simulink model "PID_Dual_Robot_DC_model_no_vision_controller"  (R2015b)
settings: Solver=ode4  StartTime=0.0  StopTime=28  FixedStep=0.01  RelTol=1e-3
InitFcn:
  | Set_Parameter_sewing_DC_model_no_vision_controller
StopFcn:
  | DrawResult_Dual
values from neighbouring files (symbols this model uses):
  b = 0.1    [Set_Parameter.m]    (also in Set_Parameter_Single.m; Set_Parameter_line_circle.m; Set_Parameter_line_circle_DC_model_no_vision_controller.m; Set_Parameter_sewing_DC_model_no_vision_controller.m)
  D = [30,30,20,20,20,20,20,20]    [Set_Parameter.m]    (also in Set_Parameter_Single.m; Set_Parameter_line_circle.m; Set_Parameter_line_circle_DC_model_no_vision_controller.m; Set_Parameter_line_circle_no_vision_controller.m = [40,40,40,30,20,30,20,20])
  I = [10,10,5,5,5,2,2,2]    [Set_Parameter.m]    (also in Set_Parameter_Single.m; Set_Parameter_line_circle.m; Set_Parameter_line_circle_DC_model_no_vision_controller.m; Set_Parameter_line_circle_no_vision_controller.m = [5,5,5,2,2,2,1,1])
  IniJointAngle_L = theta_L    [Set_Parameter.m]    (also in Set_Parameter_Single.m; Set_Parameter_line_circle.m; Set_Parameter_line_circle_DC_model_no_vision_controller.m; Set_Parameter_line_circle_no_vision_controller.m)
  IniJointAngle_R = theta_R    [Set_Parameter.m]    (also in Set_Parameter_Single.m; Set_Parameter_line_circle.m; Set_Parameter_line_circle_DC_model_no_vision_controller.m; Set_Parameter_line_circle_no_vision_controller.m)
  J = [0.016,0.016,0.012,0.012,0.01,0.01,0.01]    [Set_Parameter.m]    (also in Set_Parameter_Single.m; Set_Parameter_line_circle.m; Set_Parameter_line_circle_DC_model_no_vision_controller.m; Set_Parameter_line_circle_no_vision_controller.m = [10,10,8,8,4,4,4])
  K = 0.01    [Set_Parameter.m]    (also in Set_Parameter_Single.m; Set_Parameter_line_circle.m; Set_Parameter_line_circle_DC_model_no_vision_controller.m; Set_Parameter_sewing_DC_model_no_vision_controller.m)
  L = 0.5    [Set_Parameter.m]    (also in Set_Parameter_Single.m; Set_Parameter_line_circle.m; Set_Parameter_line_circle_DC_model_no_vision_controller.m; Set_Parameter_sewing_DC_model_no_vision_controller.m)
  P = [60,60,50,50,30,30,20,20]    [Set_Parameter.m]    (also in Set_Parameter_Single.m; Set_Parameter_line_circle.m; Set_Parameter_line_circle_DC_model_no_vision_controller.m = [120,120,100,100,60,60,40,40]; Set_Parameter_line_circle_no_vision_controller.m = [350,100,300,150,50,100,20,20])
  R = R_z1x2y3(PoseAngle(1),PoseAngle(2),PoseAngle(3))    [IK_7DOF_FB7roll.m]    (also in Set_Parameter.m = 1; Set_Parameter_Single.m = 1; Set_Parameter_line_circle.m = 1; Set_Parameter_line_circle_DC_model_no_vision_controller.m = 1)
settings Model: Creator=User  LastModifiedBy=User

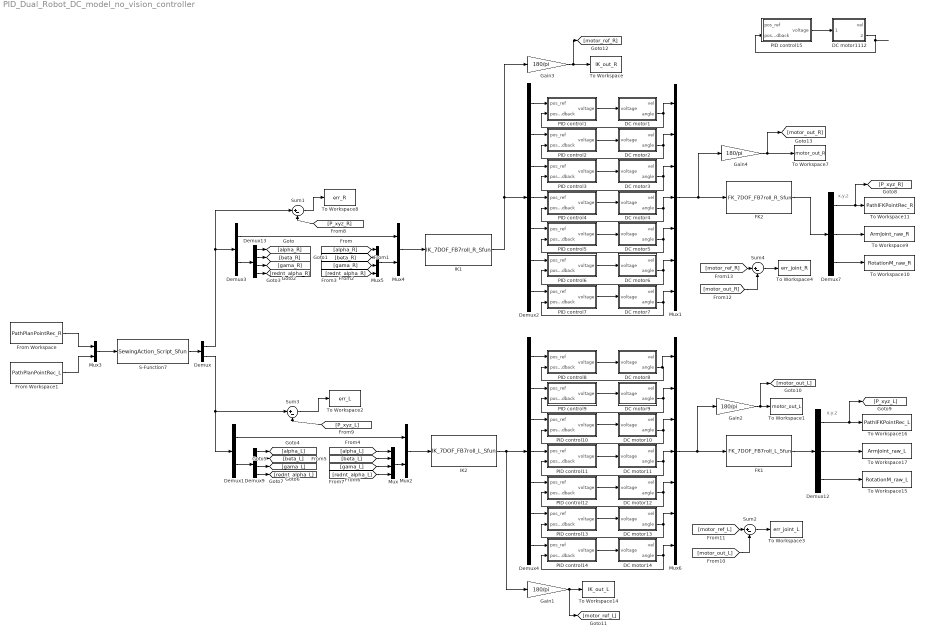
== system PID_Dual_Robot_DC_model_no_vision_controller ==
  note: x,y,z
  note: x,y,z
  DC motor1 : Subsystem
  DC motor10 : Subsystem
  DC motor11 : Subsystem
  DC motor1112 : Subsystem
  DC motor12 : Subsystem
  DC motor13 : Subsystem
  DC motor14 : Subsystem
  DC motor2 : Subsystem
  DC motor3 : Subsystem
  DC motor4 : Subsystem
  DC motor5 : Subsystem
  DC motor6 : Subsystem
  DC motor7 : Subsystem
  DC motor8 : Subsystem
  DC motor9 : Subsystem
  Demux : Demux  Outputs=[7,7]
  Demux1 : Demux  Outputs=[3,4]
  Demux12 : Demux  Outputs=[7,30,9]
  Demux13 : Demux
  Demux2 : Demux  Outputs=7
  Demux3 : Demux  Outputs=[3,4]
  Demux4 : Demux  Outputs=7
  Demux7 : Demux  Outputs=[7,30,9]
  Demux9 : Demux
  FK1 : S-Function  FunctionName=FK_7DOF_FB7roll_L_Sfun  SFunctionDeploymentMode=off  EnableBusSupport=off
  FK2 : S-Function  FunctionName=FK_7DOF_FB7roll_R_Sfun  SFunctionDeploymentMode=off  EnableBusSupport=off
  From Workspace : FromWorkspace  VariableName=PathPlanPointRec_R  SampleTime=0
  From Workspace1 : FromWorkspace  VariableName=PathPlanPointRec_L  SampleTime=0
  Gain{1..4} (4 alike) : Gain  Gain=180/pi
  IK1 : S-Function  FunctionName=IK_7DOF_FB7roll_R_Sfun  SFunctionDeploymentMode=off  EnableBusSupport=off
  IK2 : S-Function  FunctionName=IK_7DOF_FB7roll_L_Sfun  SFunctionDeploymentMode=off  EnableBusSupport=off
  Mux : Mux
  Mux1 : Mux  Inputs=7
  Mux2 : Mux  Inputs=[3,4]
  Mux3 : Mux  Inputs=[7,7]
  Mux4 : Mux  Inputs=[3,4]
  Mux5 : Mux
  Mux6 : Mux  Inputs=7
  PID control1 : Subsystem
  PID control10 : Subsystem
  PID control11 : Subsystem
  PID control12 : Subsystem
  PID control13 : Subsystem
  PID control14 : Subsystem
  PID control15 : Subsystem
  PID control2 : Subsystem
  PID control3 : Subsystem
  PID control4 : Subsystem
  PID control5 : Subsystem
  PID control6 : Subsystem
  PID control7 : Subsystem
  PID control8 : Subsystem
  PID control9 : Subsystem
  S-Function7 : S-Function  FunctionName=SewingAction_Script_Sfun  SFunctionDeploymentMode=off  EnableBusSupport=off
  Sum{1..4} (4 alike) : Sum  Inputs=|+-
  To Workspace : ToWorkspace  VariableName=IK_out_R  SaveFormat=Timeseries  SampleTime=-1
  To Workspace1 : ToWorkspace  VariableName=motor_out_L  SaveFormat=Timeseries  SampleTime=-1
  To Workspace10 : ToWorkspace  VariableName=RotationM_raw_R  SaveFormat=Timeseries  SampleTime=-1
  To Workspace11 : ToWorkspace  VariableName=PathIFKPointRec_R  SaveFormat=Timeseries  SampleTime=-1
  To Workspace14 : ToWorkspace  VariableName=IK_out_L  SaveFormat=Timeseries  SampleTime=-1
  To Workspace15 : ToWorkspace  VariableName=RotationM_raw_L  SaveFormat=Timeseries  SampleTime=-1
  To Workspace16 : ToWorkspace  VariableName=PathIFKPointRec_L  SaveFormat=Timeseries  SampleTime=-1
  To Workspace17 : ToWorkspace  VariableName=ArmJoint_raw_L  SaveFormat=Timeseries  SampleTime=-1
  To Workspace2 : ToWorkspace  VariableName=err_L  SaveFormat=Timeseries  SampleTime=-1
  To Workspace3 : ToWorkspace  VariableName=err_joint_L  SaveFormat=Timeseries  SampleTime=-1
  To Workspace4 : ToWorkspace  VariableName=err_joint_R  SaveFormat=Timeseries  SampleTime=-1
  To Workspace7 : ToWorkspace  VariableName=motor_out_R  SaveFormat=Timeseries  SampleTime=-1
  To Workspace8 : ToWorkspace  VariableName=err_R  SaveFormat=Timeseries  SampleTime=-1
  To Workspace9 : ToWorkspace  VariableName=ArmJoint_raw_R  SaveFormat=Timeseries  SampleTime=-1
  wires:
  Gain3/1 -> [motor_ref_R], To Workspace/1
  Gain4/1 -> [motor_out_R], To Workspace7/1
  Demux2/1 -> PID control1/1("pos_ref ")
  IK1/1 -> Demux2/1, Gain3/1
  Mux1/1 -> Gain4/1, FK2/1
  Mux4/1 -> IK1/1
  FK2/1 -> Demux7/1
  Demux7/1 -> To Workspace11/1, [P_xyz_R]
  Demux7/2 -> To Workspace9/1
  Demux7/3 -> To Workspace10/1
  S-Function7/1 -> Demux/1
  Demux/1 -> Sum1/1, Demux3/1
  Demux/2 -> Sum3/1, Demux1/1
  Demux9/1 -> [alpha_L]
  Demux9/2 -> [beta_L]
  Demux9/3 -> [gama_L]
  Demux9/4 -> [rednt_alpha_L]
  Demux1/2 -> Demux9/1
  [alpha_L] -> Mux/1
  [beta_L] -> Mux/2
  [gama_L] -> Mux/3
  [rednt_alpha_L] -> Mux/4
  Mux/1 -> Mux2/2
  Gain1/1 -> [motor_ref_L], To Workspace14/1
  IK2/1 -> Gain1/1, Demux4/1
  FK1/1 -> Demux12/1
  Demux12/2 -> To Workspace17/1
  Demux12/1 -> To Workspace16/1, [P_xyz_L]
  Demux12/3 -> To Workspace15/1
  Demux3/2 -> Demux13/1
  Demux13/2 -> [beta_R]
  Demux13/3 -> [gama_R]
  Demux13/4 -> [rednt_alpha_R]
  Gain2/1 -> [motor_out_L], To Workspace1/1
  Mux3/1 -> S-Function7/1
  From Workspace/1 -> Mux3/1
  From Workspace1/1 -> Mux3/2
  Mux2/1 -> IK2/1
  Mux5/1 -> Mux4/2
  [alpha_R] -> Mux5/1
  [beta_R] -> Mux5/2
  [gama_R] -> Mux5/3
  [rednt_alpha_R] -> Mux5/4
  Demux13/1 -> [alpha_R]
  PID control1/1(voltage) -> DC motor1/1(voltage)
  DC motor1/2(angle) -> Mux1/1, PID control1/2(pos_feedback)
  PID control2/1(voltage) -> DC motor2/1(voltage)
  DC motor2/2(angle) -> Mux1/2, PID control2/2(pos_feedback)
  Demux2/2 -> PID control2/1("pos_ref ")
  PID control3/1(voltage) -> DC motor3/1(voltage)
  DC motor3/2(angle) -> PID control3/2(pos_feedback), Mux1/3
  Demux2/3 -> PID control3/1("pos_ref ")
  PID control4/1(voltage) -> DC motor4/1(voltage)
  DC motor4/2(angle) -> PID control4/2(pos_feedback), Mux1/4
  Demux2/4 -> PID control4/1("pos_ref ")
  PID control5/1(voltage) -> DC motor5/1(voltage)
  DC motor5/2(angle) -> PID control5/2(pos_feedback), Mux1/5
  Demux2/5 -> PID control5/1("pos_ref ")
  PID control6/1(voltage) -> DC motor6/1(voltage)
  DC motor6/2(angle) -> PID control6/2(pos_feedback), Mux1/6
  Demux2/6 -> PID control6/1("pos_ref ")
  PID control7/1(voltage) -> DC motor7/1(voltage)
  DC motor7/2(angle) -> PID control7/2(pos_feedback), Mux1/7
  Demux2/7 -> PID control7/1("pos_ref ")
  Demux4/1 -> PID control8/1("pos_ref ")
  PID control8/1(voltage) -> DC motor8/1(voltage)
  DC motor8/2(angle) -> Mux6/1, PID control8/2(pos_feedback)
  PID control9/1(voltage) -> DC motor9/1(voltage)
  DC motor9/2(angle) -> PID control9/2(pos_feedback), Mux6/2
  Demux4/2 -> PID control9/1("pos_ref ")
  PID control10/1(voltage) -> DC motor10/1(voltage)
  DC motor10/2(angle) -> Mux6/3, PID control10/2(pos_feedback)
  Demux4/3 -> PID control10/1("pos_ref ")
  PID control11/1(voltage) -> DC motor11/1(voltage)
  DC motor11/2(angle) -> Mux6/4, PID control11/2(pos_feedback)
  Demux4/4 -> PID control11/1("pos_ref ")
  PID control12/1(voltage) -> DC motor12/1(voltage)
  DC motor12/2(angle) -> PID control12/2(pos_feedback), Mux6/5
  Demux4/5 -> PID control12/1("pos_ref ")
  PID control13/1(voltage) -> DC motor13/1(voltage)
  DC motor13/2(angle) -> PID control13/2(pos_feedback), Mux6/6
  Demux4/6 -> PID control13/1("pos_ref ")
  PID control14/1(voltage) -> DC motor14/1(voltage)
  DC motor14/2(angle) -> PID control14/2(pos_feedback), Mux6/7
  Demux4/7 -> PID control14/1("pos_ref ")
  Mux6/1 -> Gain2/1, FK1/1
  Demux3/1 -> Mux4/1
  [P_xyz_R] -> Sum1/2
  Sum1/1 -> To Workspace8/1
  Demux1/1 -> Mux2/1
  Sum3/1 -> To Workspace2/1
  [P_xyz_L] -> Sum3/2
  Sum2/1 -> To Workspace3/1
  [motor_out_L] -> Sum2/2
  [motor_ref_L] -> Sum2/1
  Sum4/1 -> To Workspace4/1
  [motor_out_R] -> Sum4/2
  [motor_ref_R] -> Sum4/1
  PID control15/1(voltage) -> DC motor1112/1(voltage)
  DC motor1112/2(angle) -> PID control15/2(pos_feedback)
  ? -> PID control15/1("pos_ref ")

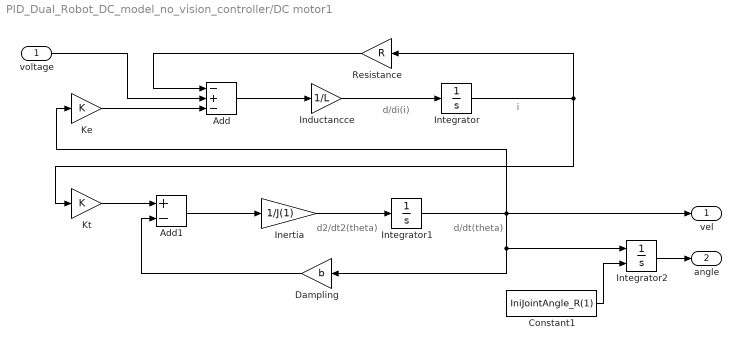
== system PID_Dual_Robot_DC_model_no_vision_controller/DC motor1 ==
  note: d/dt(theta)
  note: d2/dt2(theta)
  note: i
  note: d/di(i)
  voltage : Inport
  Add : Sum  Inputs=-+-
  Add1 : Sum  Inputs=+-
  Constant1 : Constant  Value=IniJointAngle_R(1)
  Dampling : Gain  Gain=b
  Inductancce : Gain  Gain=1/L
  Inertia : Gain  Gain=1/J(1)
  Integrator : Integrator
  Integrator1 : Integrator
  Integrator2 : Integrator  InitialConditionSource=external
  Ke : Gain  Gain=K
  Kt : Gain  Gain=K
  Resistance : Gain  Gain=R
  vel : Outport
  angle : Outport  Port=2
  wires:
  Resistance/1 -> Add/1
  Add/1 -> Inductancce/1
  Inductancce/1 -> Integrator/1
  Inertia/1 -> Integrator1/1
  Kt/1 -> Add1/1
  Add1/1 -> Inertia/1
  Integrator/1 -> Kt/1, Resistance/1
  voltage/1 -> Add/2
  Dampling/1 -> Add1/2
  Integrator1/1 -> vel/1, Ke/1, Dampling/1, Integrator2/1
  Ke/1 -> Add/3
  Constant1/1 -> Integrator2/2
  Integrator2/1 -> angle/1

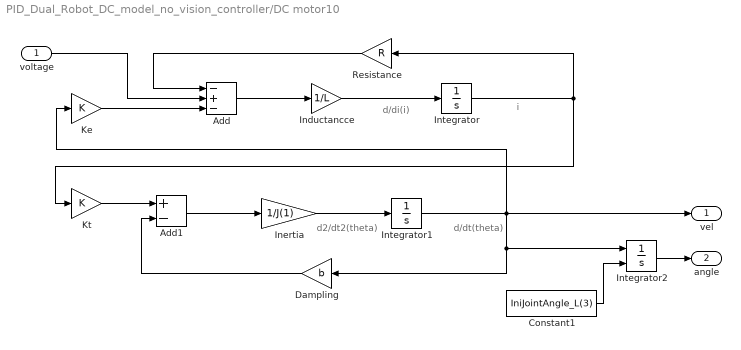
== system PID_Dual_Robot_DC_model_no_vision_controller/DC motor10 ==
  note: d/dt(theta)
  note: d2/dt2(theta)
  note: i
  note: d/di(i)
  voltage : Inport
  Add : Sum  Inputs=-+-
  Add1 : Sum  Inputs=+-
  Constant1 : Constant  Value=IniJointAngle_L(3)
  Dampling : Gain  Gain=b
  Inductancce : Gain  Gain=1/L
  Inertia : Gain  Gain=1/J(1)
  Integrator : Integrator
  Integrator1 : Integrator
  Integrator2 : Integrator  InitialConditionSource=external
  Ke : Gain  Gain=K
  Kt : Gain  Gain=K
  Resistance : Gain  Gain=R
  vel : Outport
  angle : Outport  Port=2
  wires:
  Resistance/1 -> Add/1
  Add/1 -> Inductancce/1
  Inductancce/1 -> Integrator/1
  Inertia/1 -> Integrator1/1
  Kt/1 -> Add1/1
  Add1/1 -> Inertia/1
  Integrator/1 -> Kt/1, Resistance/1
  voltage/1 -> Add/2
  Dampling/1 -> Add1/2
  Integrator1/1 -> vel/1, Ke/1, Dampling/1, Integrator2/1
  Ke/1 -> Add/3
  Constant1/1 -> Integrator2/2
  Integrator2/1 -> angle/1

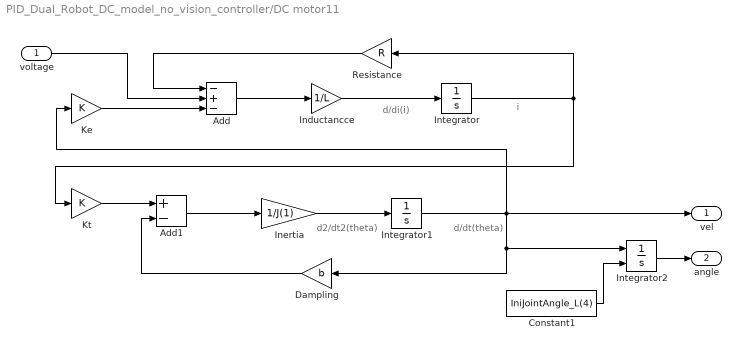
== system PID_Dual_Robot_DC_model_no_vision_controller/DC motor11 ==
  note: d/dt(theta)
  note: d2/dt2(theta)
  note: i
  note: d/di(i)
  voltage : Inport
  Add : Sum  Inputs=-+-
  Add1 : Sum  Inputs=+-
  Constant1 : Constant  Value=IniJointAngle_L(4)
  Dampling : Gain  Gain=b
  Inductancce : Gain  Gain=1/L
  Inertia : Gain  Gain=1/J(1)
  Integrator : Integrator
  Integrator1 : Integrator
  Integrator2 : Integrator  InitialConditionSource=external
  Ke : Gain  Gain=K
  Kt : Gain  Gain=K
  Resistance : Gain  Gain=R
  vel : Outport
  angle : Outport  Port=2
  wires:
  Resistance/1 -> Add/1
  Add/1 -> Inductancce/1
  Inductancce/1 -> Integrator/1
  Inertia/1 -> Integrator1/1
  Kt/1 -> Add1/1
  Add1/1 -> Inertia/1
  Integrator/1 -> Kt/1, Resistance/1
  voltage/1 -> Add/2
  Dampling/1 -> Add1/2
  Integrator1/1 -> vel/1, Ke/1, Dampling/1, Integrator2/1
  Ke/1 -> Add/3
  Constant1/1 -> Integrator2/2
  Integrator2/1 -> angle/1

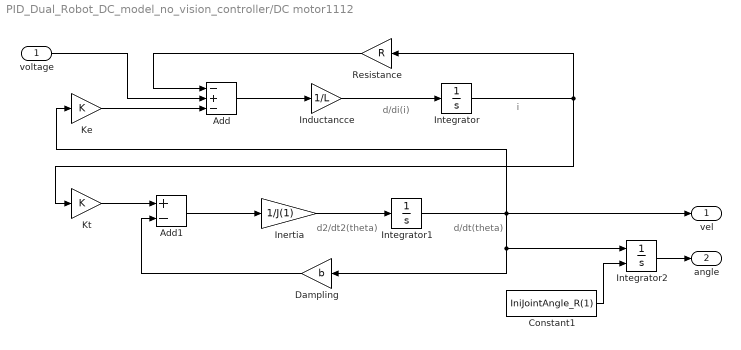
== system PID_Dual_Robot_DC_model_no_vision_controller/DC motor1112 ==
  note: d/dt(theta)
  note: d2/dt2(theta)
  note: i
  note: d/di(i)
  voltage : Inport
  Add : Sum  Inputs=-+-
  Add1 : Sum  Inputs=+-
  Constant1 : Constant  Value=IniJointAngle_R(1)
  Dampling : Gain  Gain=b
  Inductancce : Gain  Gain=1/L
  Inertia : Gain  Gain=1/J(1)
  Integrator : Integrator
  Integrator1 : Integrator
  Integrator2 : Integrator  InitialConditionSource=external
  Ke : Gain  Gain=K
  Kt : Gain  Gain=K
  Resistance : Gain  Gain=R
  vel : Outport
  angle : Outport  Port=2
  wires:
  Resistance/1 -> Add/1
  Add/1 -> Inductancce/1
  Inductancce/1 -> Integrator/1
  Inertia/1 -> Integrator1/1
  Kt/1 -> Add1/1
  Add1/1 -> Inertia/1
  Integrator/1 -> Kt/1, Resistance/1
  voltage/1 -> Add/2
  Dampling/1 -> Add1/2
  Integrator1/1 -> vel/1, Ke/1, Dampling/1, Integrator2/1
  Ke/1 -> Add/3
  Constant1/1 -> Integrator2/2
  Integrator2/1 -> angle/1

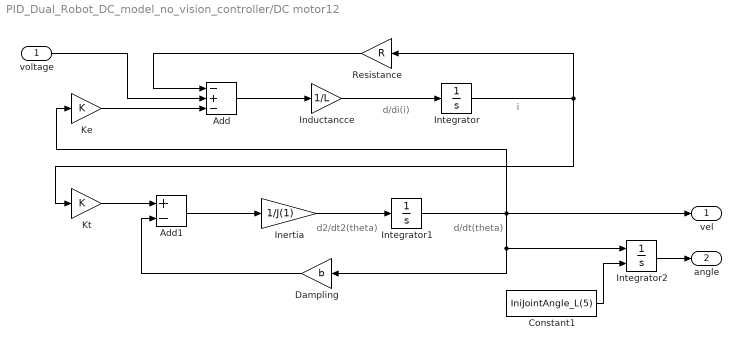
== system PID_Dual_Robot_DC_model_no_vision_controller/DC motor12 ==
  note: d/dt(theta)
  note: d2/dt2(theta)
  note: i
  note: d/di(i)
  voltage : Inport
  Add : Sum  Inputs=-+-
  Add1 : Sum  Inputs=+-
  Constant1 : Constant  Value=IniJointAngle_L(5)
  Dampling : Gain  Gain=b
  Inductancce : Gain  Gain=1/L
  Inertia : Gain  Gain=1/J(1)
  Integrator : Integrator
  Integrator1 : Integrator
  Integrator2 : Integrator  InitialConditionSource=external
  Ke : Gain  Gain=K
  Kt : Gain  Gain=K
  Resistance : Gain  Gain=R
  vel : Outport
  angle : Outport  Port=2
  wires:
  Resistance/1 -> Add/1
  Add/1 -> Inductancce/1
  Inductancce/1 -> Integrator/1
  Inertia/1 -> Integrator1/1
  Kt/1 -> Add1/1
  Add1/1 -> Inertia/1
  Integrator/1 -> Kt/1, Resistance/1
  voltage/1 -> Add/2
  Dampling/1 -> Add1/2
  Integrator1/1 -> vel/1, Ke/1, Dampling/1, Integrator2/1
  Ke/1 -> Add/3
  Constant1/1 -> Integrator2/2
  Integrator2/1 -> angle/1

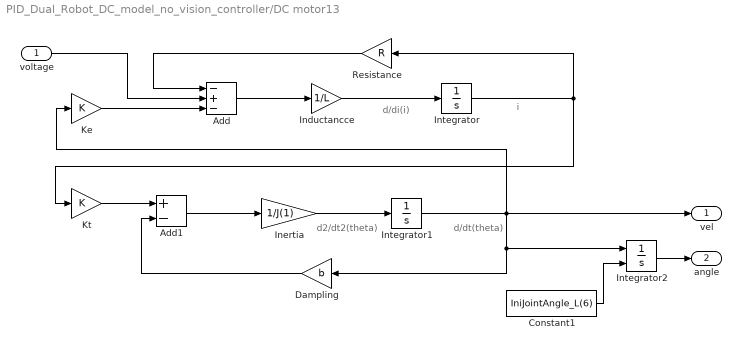
== system PID_Dual_Robot_DC_model_no_vision_controller/DC motor13 ==
  note: d/dt(theta)
  note: d2/dt2(theta)
  note: i
  note: d/di(i)
  voltage : Inport
  Add : Sum  Inputs=-+-
  Add1 : Sum  Inputs=+-
  Constant1 : Constant  Value=IniJointAngle_L(6)
  Dampling : Gain  Gain=b
  Inductancce : Gain  Gain=1/L
  Inertia : Gain  Gain=1/J(1)
  Integrator : Integrator
  Integrator1 : Integrator
  Integrator2 : Integrator  InitialConditionSource=external
  Ke : Gain  Gain=K
  Kt : Gain  Gain=K
  Resistance : Gain  Gain=R
  vel : Outport
  angle : Outport  Port=2
  wires:
  Resistance/1 -> Add/1
  Add/1 -> Inductancce/1
  Inductancce/1 -> Integrator/1
  Inertia/1 -> Integrator1/1
  Kt/1 -> Add1/1
  Add1/1 -> Inertia/1
  Integrator/1 -> Kt/1, Resistance/1
  voltage/1 -> Add/2
  Dampling/1 -> Add1/2
  Integrator1/1 -> vel/1, Ke/1, Dampling/1, Integrator2/1
  Ke/1 -> Add/3
  Constant1/1 -> Integrator2/2
  Integrator2/1 -> angle/1

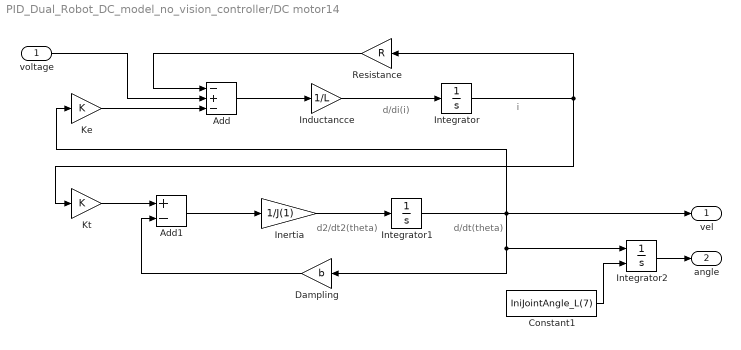
== system PID_Dual_Robot_DC_model_no_vision_controller/DC motor14 ==
  note: d/dt(theta)
  note: d2/dt2(theta)
  note: i
  note: d/di(i)
  voltage : Inport
  Add : Sum  Inputs=-+-
  Add1 : Sum  Inputs=+-
  Constant1 : Constant  Value=IniJointAngle_L(7)
  Dampling : Gain  Gain=b
  Inductancce : Gain  Gain=1/L
  Inertia : Gain  Gain=1/J(1)
  Integrator : Integrator
  Integrator1 : Integrator
  Integrator2 : Integrator  InitialConditionSource=external
  Ke : Gain  Gain=K
  Kt : Gain  Gain=K
  Resistance : Gain  Gain=R
  vel : Outport
  angle : Outport  Port=2
  wires:
  Resistance/1 -> Add/1
  Add/1 -> Inductancce/1
  Inductancce/1 -> Integrator/1
  Inertia/1 -> Integrator1/1
  Kt/1 -> Add1/1
  Add1/1 -> Inertia/1
  Integrator/1 -> Kt/1, Resistance/1
  voltage/1 -> Add/2
  Dampling/1 -> Add1/2
  Integrator1/1 -> vel/1, Ke/1, Dampling/1, Integrator2/1
  Ke/1 -> Add/3
  Constant1/1 -> Integrator2/2
  Integrator2/1 -> angle/1

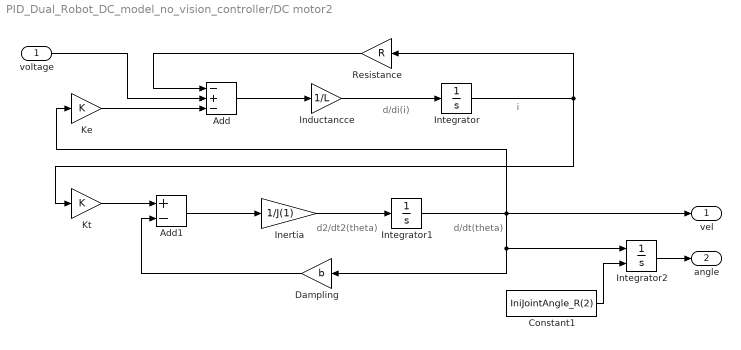
== system PID_Dual_Robot_DC_model_no_vision_controller/DC motor2 ==
  note: d/dt(theta)
  note: d2/dt2(theta)
  note: i
  note: d/di(i)
  voltage : Inport
  Add : Sum  Inputs=-+-
  Add1 : Sum  Inputs=+-
  Constant1 : Constant  Value=IniJointAngle_R(2)
  Dampling : Gain  Gain=b
  Inductancce : Gain  Gain=1/L
  Inertia : Gain  Gain=1/J(1)
  Integrator : Integrator
  Integrator1 : Integrator
  Integrator2 : Integrator  InitialConditionSource=external
  Ke : Gain  Gain=K
  Kt : Gain  Gain=K
  Resistance : Gain  Gain=R
  vel : Outport
  angle : Outport  Port=2
  wires:
  Resistance/1 -> Add/1
  Add/1 -> Inductancce/1
  Inductancce/1 -> Integrator/1
  Inertia/1 -> Integrator1/1
  Kt/1 -> Add1/1
  Add1/1 -> Inertia/1
  Integrator/1 -> Kt/1, Resistance/1
  voltage/1 -> Add/2
  Dampling/1 -> Add1/2
  Integrator1/1 -> vel/1, Ke/1, Dampling/1, Integrator2/1
  Ke/1 -> Add/3
  Constant1/1 -> Integrator2/2
  Integrator2/1 -> angle/1

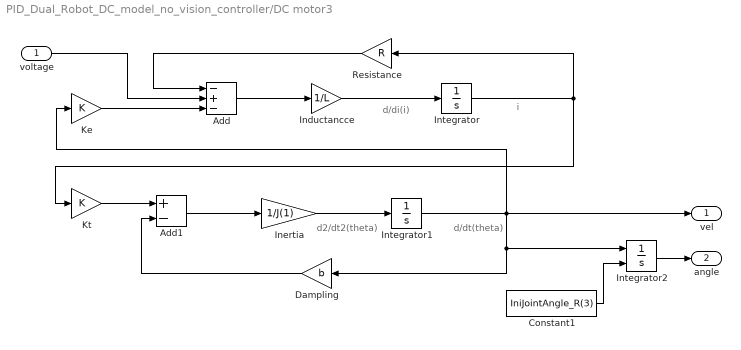
== system PID_Dual_Robot_DC_model_no_vision_controller/DC motor3 ==
  note: d/dt(theta)
  note: d2/dt2(theta)
  note: i
  note: d/di(i)
  voltage : Inport
  Add : Sum  Inputs=-+-
  Add1 : Sum  Inputs=+-
  Constant1 : Constant  Value=IniJointAngle_R(3)
  Dampling : Gain  Gain=b
  Inductancce : Gain  Gain=1/L
  Inertia : Gain  Gain=1/J(1)
  Integrator : Integrator
  Integrator1 : Integrator
  Integrator2 : Integrator  InitialConditionSource=external
  Ke : Gain  Gain=K
  Kt : Gain  Gain=K
  Resistance : Gain  Gain=R
  vel : Outport
  angle : Outport  Port=2
  wires:
  Resistance/1 -> Add/1
  Add/1 -> Inductancce/1
  Inductancce/1 -> Integrator/1
  Inertia/1 -> Integrator1/1
  Kt/1 -> Add1/1
  Add1/1 -> Inertia/1
  Integrator/1 -> Kt/1, Resistance/1
  voltage/1 -> Add/2
  Dampling/1 -> Add1/2
  Integrator1/1 -> vel/1, Ke/1, Dampling/1, Integrator2/1
  Ke/1 -> Add/3
  Constant1/1 -> Integrator2/2
  Integrator2/1 -> angle/1

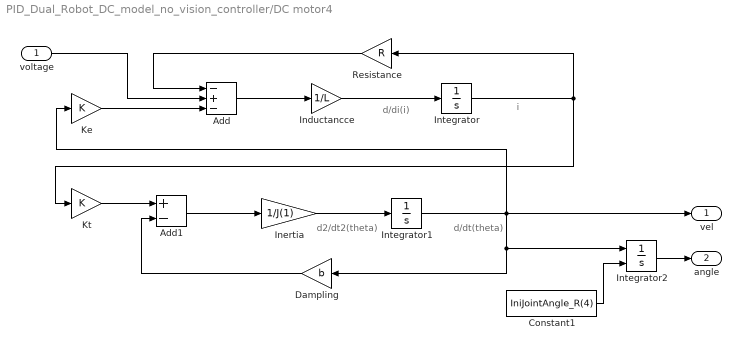
== system PID_Dual_Robot_DC_model_no_vision_controller/DC motor4 ==
  note: d/dt(theta)
  note: d2/dt2(theta)
  note: i
  note: d/di(i)
  voltage : Inport
  Add : Sum  Inputs=-+-
  Add1 : Sum  Inputs=+-
  Constant1 : Constant  Value=IniJointAngle_R(4)
  Dampling : Gain  Gain=b
  Inductancce : Gain  Gain=1/L
  Inertia : Gain  Gain=1/J(1)
  Integrator : Integrator
  Integrator1 : Integrator
  Integrator2 : Integrator  InitialConditionSource=external
  Ke : Gain  Gain=K
  Kt : Gain  Gain=K
  Resistance : Gain  Gain=R
  vel : Outport
  angle : Outport  Port=2
  wires:
  Resistance/1 -> Add/1
  Add/1 -> Inductancce/1
  Inductancce/1 -> Integrator/1
  Inertia/1 -> Integrator1/1
  Kt/1 -> Add1/1
  Add1/1 -> Inertia/1
  Integrator/1 -> Kt/1, Resistance/1
  voltage/1 -> Add/2
  Dampling/1 -> Add1/2
  Integrator1/1 -> vel/1, Ke/1, Dampling/1, Integrator2/1
  Ke/1 -> Add/3
  Constant1/1 -> Integrator2/2
  Integrator2/1 -> angle/1

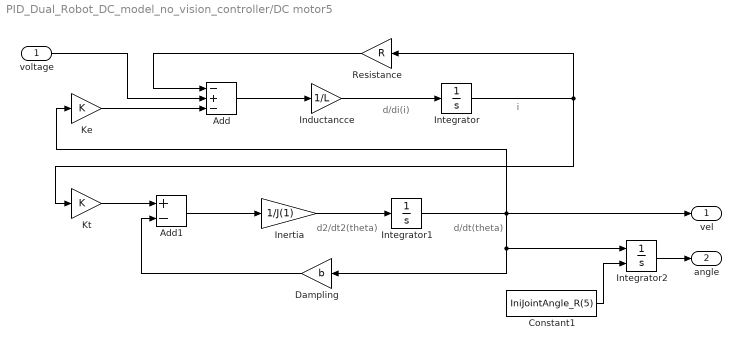
== system PID_Dual_Robot_DC_model_no_vision_controller/DC motor5 ==
  note: d/dt(theta)
  note: d2/dt2(theta)
  note: i
  note: d/di(i)
  voltage : Inport
  Add : Sum  Inputs=-+-
  Add1 : Sum  Inputs=+-
  Constant1 : Constant  Value=IniJointAngle_R(5)
  Dampling : Gain  Gain=b
  Inductancce : Gain  Gain=1/L
  Inertia : Gain  Gain=1/J(1)
  Integrator : Integrator
  Integrator1 : Integrator
  Integrator2 : Integrator  InitialConditionSource=external
  Ke : Gain  Gain=K
  Kt : Gain  Gain=K
  Resistance : Gain  Gain=R
  vel : Outport
  angle : Outport  Port=2
  wires:
  Resistance/1 -> Add/1
  Add/1 -> Inductancce/1
  Inductancce/1 -> Integrator/1
  Inertia/1 -> Integrator1/1
  Kt/1 -> Add1/1
  Add1/1 -> Inertia/1
  Integrator/1 -> Kt/1, Resistance/1
  voltage/1 -> Add/2
  Dampling/1 -> Add1/2
  Integrator1/1 -> vel/1, Ke/1, Dampling/1, Integrator2/1
  Ke/1 -> Add/3
  Constant1/1 -> Integrator2/2
  Integrator2/1 -> angle/1

== system PID_Dual_Robot_DC_model_no_vision_controller/DC motor6 ==
  note: d/dt(theta)
  note: d2/dt2(theta)
  note: i
  note: d/di(i)
  voltage : Inport
  Add : Sum  Inputs=-+-
  Add1 : Sum  Inputs=+-
  Constant1 : Constant  Value=IniJointAngle_R(6)
  Dampling : Gain  Gain=b
  Inductancce : Gain  Gain=1/L
  Inertia : Gain  Gain=1/J(1)
  Integrator : Integrator
  Integrator1 : Integrator
  Integrator2 : Integrator  InitialConditionSource=external
  Ke : Gain  Gain=K
  Kt : Gain  Gain=K
  Resistance : Gain  Gain=R
  vel : Outport
  angle : Outport  Port=2
  wires:
  Resistance/1 -> Add/1
  Add/1 -> Inductancce/1
  Inductancce/1 -> Integrator/1
  Inertia/1 -> Integrator1/1
  Kt/1 -> Add1/1
  Add1/1 -> Inertia/1
  Integrator/1 -> Kt/1, Resistance/1
  voltage/1 -> Add/2
  Dampling/1 -> Add1/2
  Integrator1/1 -> vel/1, Ke/1, Dampling/1, Integrator2/1
  Ke/1 -> Add/3
  Constant1/1 -> Integrator2/2
  Integrator2/1 -> angle/1

== system PID_Dual_Robot_DC_model_no_vision_controller/DC motor7 ==
  note: d/dt(theta)
  note: d2/dt2(theta)
  note: i
  note: d/di(i)
  voltage : Inport
  Add : Sum  Inputs=-+-
  Add1 : Sum  Inputs=+-
  Constant1 : Constant  Value=IniJointAngle_R(7)
  Dampling : Gain  Gain=b
  Inductancce : Gain  Gain=1/L
  Inertia : Gain  Gain=1/J(1)
  Integrator : Integrator
  Integrator1 : Integrator
  Integrator2 : Integrator  InitialConditionSource=external
  Ke : Gain  Gain=K
  Kt : Gain  Gain=K
  Resistance : Gain  Gain=R
  vel : Outport
  angle : Outport  Port=2
  wires:
  Resistance/1 -> Add/1
  Add/1 -> Inductancce/1
  Inductancce/1 -> Integrator/1
  Inertia/1 -> Integrator1/1
  Kt/1 -> Add1/1
  Add1/1 -> Inertia/1
  Integrator/1 -> Kt/1, Resistance/1
  voltage/1 -> Add/2
  Dampling/1 -> Add1/2
  Integrator1/1 -> vel/1, Ke/1, Dampling/1, Integrator2/1
  Ke/1 -> Add/3
  Constant1/1 -> Integrator2/2
  Integrator2/1 -> angle/1

== system PID_Dual_Robot_DC_model_no_vision_controller/DC motor8 ==
  note: d/dt(theta)
  note: d2/dt2(theta)
  note: i
  note: d/di(i)
  voltage : Inport
  Add : Sum  Inputs=-+-
  Add1 : Sum  Inputs=+-
  Constant1 : Constant  Value=IniJointAngle_L(1)
  Dampling : Gain  Gain=b
  Inductancce : Gain  Gain=1/L
  Inertia : Gain  Gain=1/J(1)
  Integrator : Integrator
  Integrator1 : Integrator
  Integrator2 : Integrator  InitialConditionSource=external
  Ke : Gain  Gain=K
  Kt : Gain  Gain=K
  Resistance : Gain  Gain=R
  vel : Outport
  angle : Outport  Port=2
  wires:
  Resistance/1 -> Add/1
  Add/1 -> Inductancce/1
  Inductancce/1 -> Integrator/1
  Inertia/1 -> Integrator1/1
  Kt/1 -> Add1/1
  Add1/1 -> Inertia/1
  Integrator/1 -> Kt/1, Resistance/1
  voltage/1 -> Add/2
  Dampling/1 -> Add1/2
  Integrator1/1 -> vel/1, Ke/1, Dampling/1, Integrator2/1
  Ke/1 -> Add/3
  Constant1/1 -> Integrator2/2
  Integrator2/1 -> angle/1

== system PID_Dual_Robot_DC_model_no_vision_controller/DC motor9 ==
  note: d/dt(theta)
  note: d2/dt2(theta)
  note: i
  note: d/di(i)
  voltage : Inport
  Add : Sum  Inputs=-+-
  Add1 : Sum  Inputs=+-
  Constant1 : Constant  Value=IniJointAngle_L(2)
  Dampling : Gain  Gain=b
  Inductancce : Gain  Gain=1/L
  Inertia : Gain  Gain=1/J(1)
  Integrator : Integrator
  Integrator1 : Integrator
  Integrator2 : Integrator  InitialConditionSource=external
  Ke : Gain  Gain=K
  Kt : Gain  Gain=K
  Resistance : Gain  Gain=R
  vel : Outport
  angle : Outport  Port=2
  wires:
  Resistance/1 -> Add/1
  Add/1 -> Inductancce/1
  Inductancce/1 -> Integrator/1
  Inertia/1 -> Integrator1/1
  Kt/1 -> Add1/1
  Add1/1 -> Inertia/1
  Integrator/1 -> Kt/1, Resistance/1
  voltage/1 -> Add/2
  Dampling/1 -> Add1/2
  Integrator1/1 -> vel/1, Ke/1, Dampling/1, Integrator2/1
  Ke/1 -> Add/3
  Constant1/1 -> Integrator2/2
  Integrator2/1 -> angle/1

== system PID_Dual_Robot_DC_model_no_vision_controller/PID control1 ==
  "pos_ref " : Inport
  pos_feedback : Inport  Port=2
  Derivative1 : Derivative
  Integrator4 : Integrator
  Kd : Gain  Gain=D(1)
  Ki : Gain  Gain=I(1)
  Kp : Gain  Gain=P(1)
  Sum3 : Sum  Inputs=|+-
  Sum5 : Sum  Inputs=+|+|+
  voltage : Outport
  wires:
  Sum5/1 -> voltage/1
  Kp/1 -> Sum5/1
  "pos_ref "/1 -> Sum3/1
  pos_feedback/1 -> Sum3/2
  Sum3/1 -> Derivative1/1, Integrator4/1, Kp/1
  Kd/1 -> Sum5/3
  Derivative1/1 -> Kd/1
  Integrator4/1 -> Ki/1
  Ki/1 -> Sum5/2

== system PID_Dual_Robot_DC_model_no_vision_controller/PID control10 ==
  "pos_ref " : Inport
  pos_feedback : Inport  Port=2
  Derivative1 : Derivative
  Integrator4 : Integrator
  Kd : Gain  Gain=D(3)
  Ki : Gain  Gain=I(3)
  Kp : Gain  Gain=P(3)
  Sum3 : Sum  Inputs=|+-
  Sum5 : Sum  Inputs=+|+|+
  voltage : Outport
  wires:
  Sum5/1 -> voltage/1
  Kp/1 -> Sum5/1
  "pos_ref "/1 -> Sum3/1
  pos_feedback/1 -> Sum3/2
  Sum3/1 -> Derivative1/1, Integrator4/1, Kp/1
  Kd/1 -> Sum5/3
  Derivative1/1 -> Kd/1
  Integrator4/1 -> Ki/1
  Ki/1 -> Sum5/2

== system PID_Dual_Robot_DC_model_no_vision_controller/PID control11 ==
  "pos_ref " : Inport
  pos_feedback : Inport  Port=2
  Derivative1 : Derivative
  Integrator4 : Integrator
  Kd : Gain  Gain=D(4)
  Ki : Gain  Gain=I(4)
  Kp : Gain  Gain=P(4)
  Sum3 : Sum  Inputs=|+-
  Sum5 : Sum  Inputs=+|+|+
  voltage : Outport
  wires:
  Sum5/1 -> voltage/1
  Kp/1 -> Sum5/1
  "pos_ref "/1 -> Sum3/1
  pos_feedback/1 -> Sum3/2
  Sum3/1 -> Derivative1/1, Integrator4/1, Kp/1
  Kd/1 -> Sum5/3
  Derivative1/1 -> Kd/1
  Integrator4/1 -> Ki/1
  Ki/1 -> Sum5/2

== system PID_Dual_Robot_DC_model_no_vision_controller/PID control12 ==
  "pos_ref " : Inport
  pos_feedback : Inport  Port=2
  Derivative1 : Derivative
  Integrator4 : Integrator
  Kd : Gain  Gain=D(5)
  Ki : Gain  Gain=I(5)
  Kp : Gain  Gain=P(5)
  Sum3 : Sum  Inputs=|+-
  Sum5 : Sum  Inputs=+|+|+
  voltage : Outport
  wires:
  Sum5/1 -> voltage/1
  Kp/1 -> Sum5/1
  "pos_ref "/1 -> Sum3/1
  pos_feedback/1 -> Sum3/2
  Sum3/1 -> Derivative1/1, Integrator4/1, Kp/1
  Kd/1 -> Sum5/3
  Derivative1/1 -> Kd/1
  Integrator4/1 -> Ki/1
  Ki/1 -> Sum5/2

== system PID_Dual_Robot_DC_model_no_vision_controller/PID control13 ==
  "pos_ref " : Inport
  pos_feedback : Inport  Port=2
  Derivative1 : Derivative
  Integrator4 : Integrator
  Kd : Gain  Gain=D(6)
  Ki : Gain  Gain=I(6)
  Kp : Gain  Gain=P(6)
  Sum3 : Sum  Inputs=|+-
  Sum5 : Sum  Inputs=+|+|+
  voltage : Outport
  wires:
  Sum5/1 -> voltage/1
  Kp/1 -> Sum5/1
  "pos_ref "/1 -> Sum3/1
  pos_feedback/1 -> Sum3/2
  Sum3/1 -> Derivative1/1, Integrator4/1, Kp/1
  Kd/1 -> Sum5/3
  Derivative1/1 -> Kd/1
  Integrator4/1 -> Ki/1
  Ki/1 -> Sum5/2

== system PID_Dual_Robot_DC_model_no_vision_controller/PID control14 ==
  "pos_ref " : Inport
  pos_feedback : Inport  Port=2
  Derivative1 : Derivative
  Integrator4 : Integrator
  Kd : Gain  Gain=D(7)
  Ki : Gain  Gain=I(7)
  Kp : Gain  Gain=P(7)
  Sum3 : Sum  Inputs=|+-
  Sum5 : Sum  Inputs=+|+|+
  voltage : Outport
  wires:
  Sum5/1 -> voltage/1
  Kp/1 -> Sum5/1
  "pos_ref "/1 -> Sum3/1
  pos_feedback/1 -> Sum3/2
  Sum3/1 -> Derivative1/1, Integrator4/1, Kp/1
  Kd/1 -> Sum5/3
  Derivative1/1 -> Kd/1
  Integrator4/1 -> Ki/1
  Ki/1 -> Sum5/2

== system PID_Dual_Robot_DC_model_no_vision_controller/PID control15 ==
  "pos_ref " : Inport
  pos_feedback : Inport  Port=2
  Derivative1 : Derivative
  Integrator4 : Integrator
  Kd : Gain  Gain=D(1)
  Ki : Gain  Gain=I(1)
  Kp : Gain  Gain=P(1)
  Sum3 : Sum  Inputs=|+-
  Sum5 : Sum  Inputs=+|+|+
  voltage : Outport
  wires:
  Sum5/1 -> voltage/1
  Kp/1 -> Sum5/1
  "pos_ref "/1 -> Sum3/1
  pos_feedback/1 -> Sum3/2
  Sum3/1 -> Derivative1/1, Integrator4/1, Kp/1
  Kd/1 -> Sum5/3
  Derivative1/1 -> Kd/1
  Integrator4/1 -> Ki/1
  Ki/1 -> Sum5/2

== system PID_Dual_Robot_DC_model_no_vision_controller/PID control2 ==
  "pos_ref " : Inport
  pos_feedback : Inport  Port=2
  Derivative1 : Derivative
  Integrator4 : Integrator
  Kd : Gain  Gain=D(2)
  Ki : Gain  Gain=I(2)
  Kp : Gain  Gain=P(2)
  Sum3 : Sum  Inputs=|+-
  Sum5 : Sum  Inputs=+|+|+
  voltage : Outport
  wires:
  Sum5/1 -> voltage/1
  Kp/1 -> Sum5/1
  "pos_ref "/1 -> Sum3/1
  pos_feedback/1 -> Sum3/2
  Sum3/1 -> Derivative1/1, Integrator4/1, Kp/1
  Kd/1 -> Sum5/3
  Derivative1/1 -> Kd/1
  Integrator4/1 -> Ki/1
  Ki/1 -> Sum5/2

== system PID_Dual_Robot_DC_model_no_vision_controller/PID control3 ==
  "pos_ref " : Inport
  pos_feedback : Inport  Port=2
  Derivative1 : Derivative
  Integrator4 : Integrator
  Kd : Gain  Gain=D(3)
  Ki : Gain  Gain=I(3)
  Kp : Gain  Gain=P(3)
  Sum3 : Sum  Inputs=|+-
  Sum5 : Sum  Inputs=+|+|+
  voltage : Outport
  wires:
  Sum5/1 -> voltage/1
  Kp/1 -> Sum5/1
  "pos_ref "/1 -> Sum3/1
  pos_feedback/1 -> Sum3/2
  Sum3/1 -> Derivative1/1, Integrator4/1, Kp/1
  Kd/1 -> Sum5/3
  Derivative1/1 -> Kd/1
  Integrator4/1 -> Ki/1
  Ki/1 -> Sum5/2

== system PID_Dual_Robot_DC_model_no_vision_controller/PID control4 ==
  "pos_ref " : Inport
  pos_feedback : Inport  Port=2
  Derivative1 : Derivative
  Integrator4 : Integrator
  Kd : Gain  Gain=D(4)
  Ki : Gain  Gain=I(4)
  Kp : Gain  Gain=P(4)
  Sum3 : Sum  Inputs=|+-
  Sum5 : Sum  Inputs=+|+|+
  voltage : Outport
  wires:
  Sum5/1 -> voltage/1
  Kp/1 -> Sum5/1
  "pos_ref "/1 -> Sum3/1
  pos_feedback/1 -> Sum3/2
  Sum3/1 -> Derivative1/1, Integrator4/1, Kp/1
  Kd/1 -> Sum5/3
  Derivative1/1 -> Kd/1
  Integrator4/1 -> Ki/1
  Ki/1 -> Sum5/2

== system PID_Dual_Robot_DC_model_no_vision_controller/PID control5 ==
  "pos_ref " : Inport
  pos_feedback : Inport  Port=2
  Derivative1 : Derivative
  Integrator4 : Integrator
  Kd : Gain  Gain=D(5)
  Ki : Gain  Gain=I(5)
  Kp : Gain  Gain=P(5)
  Sum3 : Sum  Inputs=|+-
  Sum5 : Sum  Inputs=+|+|+
  voltage : Outport
  wires:
  Sum5/1 -> voltage/1
  Kp/1 -> Sum5/1
  "pos_ref "/1 -> Sum3/1
  pos_feedback/1 -> Sum3/2
  Sum3/1 -> Derivative1/1, Integrator4/1, Kp/1
  Kd/1 -> Sum5/3
  Derivative1/1 -> Kd/1
  Integrator4/1 -> Ki/1
  Ki/1 -> Sum5/2

== system PID_Dual_Robot_DC_model_no_vision_controller/PID control6 ==
  "pos_ref " : Inport
  pos_feedback : Inport  Port=2
  Derivative1 : Derivative
  Integrator4 : Integrator
  Kd : Gain  Gain=D(6)
  Ki : Gain  Gain=I(6)
  Kp : Gain  Gain=P(6)
  Sum3 : Sum  Inputs=|+-
  Sum5 : Sum  Inputs=+|+|+
  voltage : Outport
  wires:
  Sum5/1 -> voltage/1
  Kp/1 -> Sum5/1
  "pos_ref "/1 -> Sum3/1
  pos_feedback/1 -> Sum3/2
  Sum3/1 -> Derivative1/1, Integrator4/1, Kp/1
  Kd/1 -> Sum5/3
  Derivative1/1 -> Kd/1
  Integrator4/1 -> Ki/1
  Ki/1 -> Sum5/2

== system PID_Dual_Robot_DC_model_no_vision_controller/PID control7 ==
  "pos_ref " : Inport
  pos_feedback : Inport  Port=2
  Derivative1 : Derivative
  Integrator4 : Integrator
  Kd : Gain  Gain=D(7)
  Ki : Gain  Gain=I(7)
  Kp : Gain  Gain=P(7)
  Sum3 : Sum  Inputs=|+-
  Sum5 : Sum  Inputs=+|+|+
  voltage : Outport
  wires:
  Sum5/1 -> voltage/1
  Kp/1 -> Sum5/1
  "pos_ref "/1 -> Sum3/1
  pos_feedback/1 -> Sum3/2
  Sum3/1 -> Derivative1/1, Integrator4/1, Kp/1
  Kd/1 -> Sum5/3
  Derivative1/1 -> Kd/1
  Integrator4/1 -> Ki/1
  Ki/1 -> Sum5/2

== system PID_Dual_Robot_DC_model_no_vision_controller/PID control8 ==
  "pos_ref " : Inport
  pos_feedback : Inport  Port=2
  Derivative1 : Derivative
  Integrator4 : Integrator
  Kd : Gain  Gain=D(1)
  Ki : Gain  Gain=I(1)
  Kp : Gain  Gain=P(1)
  Sum3 : Sum  Inputs=|+-
  Sum5 : Sum  Inputs=+|+|+
  voltage : Outport
  wires:
  Sum5/1 -> voltage/1
  Kp/1 -> Sum5/1
  "pos_ref "/1 -> Sum3/1
  pos_feedback/1 -> Sum3/2
  Sum3/1 -> Derivative1/1, Integrator4/1, Kp/1
  Kd/1 -> Sum5/3
  Derivative1/1 -> Kd/1
  Integrator4/1 -> Ki/1
  Ki/1 -> Sum5/2

== system PID_Dual_Robot_DC_model_no_vision_controller/PID control9 ==
  "pos_ref " : Inport
  pos_feedback : Inport  Port=2
  Derivative1 : Derivative
  Integrator4 : Integrator
  Kd : Gain  Gain=D(2)
  Ki : Gain  Gain=I(2)
  Kp : Gain  Gain=P(2)
  Sum3 : Sum  Inputs=|+-
  Sum5 : Sum  Inputs=+|+|+
  voltage : Outport
  wires:
  Sum5/1 -> voltage/1
  Kp/1 -> Sum5/1
  "pos_ref "/1 -> Sum3/1
  pos_feedback/1 -> Sum3/2
  Sum3/1 -> Derivative1/1, Integrator4/1, Kp/1
  Kd/1 -> Sum5/3
  Derivative1/1 -> Kd/1
  Integrator4/1 -> Ki/1
  Ki/1 -> Sum5/2
